simulink model "TWFL_V2"  (R2025b)
settings: Solver=daessc  StartTime=0.0  StopTime=15  RelTol=1e-3
values from neighbouring files (symbols this model uses):
  g = 9.81    [model_simplified.m]    (also in robotParams.m)
  g_fork = 2*pi*3    (= 18.8495559215)    [robotParams.m]
  g_lift = 2*pi*5    (= 31.4159265359)    [robotParams.m]
  g_reac = 2*pi*1    (= 6.28318530718)    [robotParams.m]
  Kd_fork = 100    [robotParams.m]
  Kd_lift = 50    [robotParams.m]
  Kp_fork = 200    [robotParams.m]
  Kp_lift = 200    [robotParams.m]
  Lx_b = 0.3    [robotParams.m]
  Lx_m = 0.1    [robotParams.m]
  Ly_b = 0.8    [robotParams.m]
  Ly_m = 0.3    [robotParams.m]
  Lz_b = 1    [robotParams.m]
  Lz_m = 1.5    [robotParams.m]
  M_arm_motor = 5    [robotParams.m]
  M_b = 16    [robotParams.m]
  M_fork_base = 2    [robotParams.m]
  M_m = 5    [robotParams.m]
  M_tooth = 1    [robotParams.m]
  M_w = 1    [robotParams.m]
  N = 40    [ocp_arm.m]    (also in ocp_simplified.m)
  r_w = 0.2    [model_simplified.m]    (also in robotParams.m)
  T_control = 1e-3    (= 0.001)    [robotParams.m]
  t_w = 0.05    [robotParams.m]
undefined symbols (not defined in the file or in its folder): dspblkCoreblockFVToolHelper, gcbh, Mn_33, Mn_44, X, Y, Z
libraries: sm_lib x49, nesl_utility x13, simulink x9, slpidlib x1, SignalEditorBlockLib x1
(part 3 of 3)

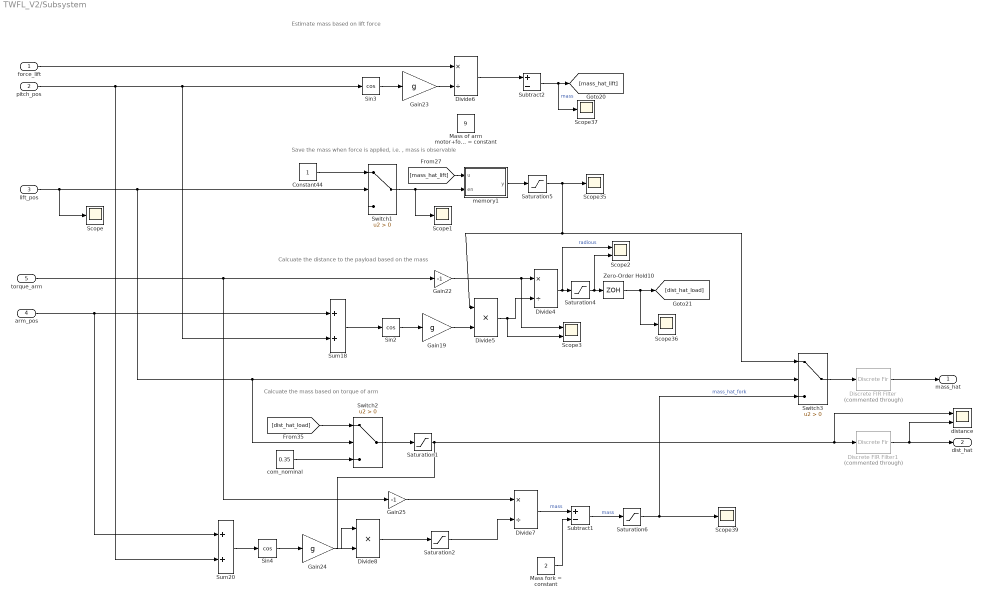
== system TWFL_V2/Subsystem ==
  note: Estimate mass based on lift force
  note: Save the mass when force is applied, i.e. , mass is observable
  note: Calcuate the distance to the payload based on the mass
  note: Calcuate the mass based on torque of arm
  force_lift : Inport
  pitch_pos : Inport  Port=2
  lift_pos : Inport  Port=3
  arm_pos : Inport  Port=4
  torque_arm : Inport  Port=5
  Constant44 : Constant
  Discrete FIR Filter : DiscreteFir  Commented=through  LoadFcn=dspblkCoreblockFVToolHelper(gcbh,'load');  Coefficients=ones(1,5000)/5000
      settings: CopyFcn=dspblkCoreblockFVToolHelper(gcbh,'copy');  DeleteFcn=dspblkCoreblockFVToolHelper(gcbh,'close');  ModelCloseFcn=dspblkCoreblockFVToolHelper(gcbh,'close');  PreSaveFcn=dspblkCoreblockFVToolHelper(gcbh,'presave');  PostSaveFcn=dspblkCoreblockFVToolHelper(gcbh,'postsave');  CloseFcn=dspblkCoreblockFVToolHelper(gcbh,'close');
  Discrete FIR Filter1 : DiscreteFir  Commented=through  LoadFcn=dspblkCoreblockFVToolHelper(gcbh,'load');  Coefficients=ones(1,500)/500
      settings: CopyFcn=dspblkCoreblockFVToolHelper(gcbh,'copy');  DeleteFcn=dspblkCoreblockFVToolHelper(gcbh,'close');  ModelCloseFcn=dspblkCoreblockFVToolHelper(gcbh,'close');  PreSaveFcn=dspblkCoreblockFVToolHelper(gcbh,'presave');  PostSaveFcn=dspblkCoreblockFVToolHelper(gcbh,'postsave');  CloseFcn=dspblkCoreblockFVToolHelper(gcbh,'close');
  Divide4 : Product  Inputs=*/
  Divide5 : Product  Inputs=**
  Divide6 : Product  Inputs=*/
  Divide7 : Product  Inputs=*/
  Divide8 : Product  Inputs=**
  Gain19 : Gain  Gain=g
  Gain22 : Gain  Gain=-1
  Gain23 : Gain  Gain=g
  Gain24 : Gain  Gain=g
  Gain25 : Gain  Gain=-1
  Mass fork = constant : Constant  Value=2
  Mass of arm motor+fork = constant : Constant  Value=9
  Saturation1 : Saturate  UpperLimit=0.6  LowerLimit=0.1
  Saturation2 : Saturate  UpperLimit=inf  LowerLimit=0.1
  Saturation4 : Saturate  UpperLimit=0.6  LowerLimit=0.1
  Saturation5 : Saturate  UpperLimit=20  LowerLimit=0.001
  Saturation6 : Saturate  UpperLimit=20  LowerLimit=0
  Scope{,1,35..37,39} (6 alike) : Scope
      Scope settings: ActiveDisplayYMinimum=0.070361077430227931  ActiveDisplayYMaximum=0.28346517515409136  DataLoggingVariableName=ScopeData8
      Scope1 settings: ActiveDisplayYMinimum=-1  ActiveDisplayYMaximum=1  DataLoggingVariableName=ScopeData23
      Scope35 settings: ActiveDisplayYMinimum=-8.2304071109691854  ActiveDisplayYMaximum=20.638497565504139  DataLoggingVariableName=ScopeData41
      Scope36 settings: ActiveDisplayYMinimum=0.4275366294753099  ActiveDisplayYMaximum=0.68738197605097551  DataLoggingVariableName=ScopeData42
      Scope37 settings: ActiveDisplayYMinimum=-38.285966258289932  ActiveDisplayYMaximum=64.906768166290135  DataLoggingVariableName=ScopeData43
      Scope39 settings: ActiveDisplayYMinimum=-0.718038981848304  ActiveDisplayYMaximum=31.278716537533729  DataLoggingVariableName=ScopeData45
  Scope2 : Scope  NumInputPorts=2
      settings: ActiveDisplayYMinimum=-736.6219251517366  ActiveDisplayYMaximum=1535.2926904846679  DataLoggingVariableName=ScopeData24
  Scope3 : Scope  NumInputPorts=2
      settings: ActiveDisplayYMinimum=69.229442757721216  ActiveDisplayYMaximum=203.32446584581058  DataLoggingVariableName=ScopeData25
  Sin2 : Trigonometry  Operator=cos
  Sin3 : Trigonometry  Operator=cos
  Sin4 : Trigonometry  Operator=cos
  Subtract1 : Sum  Inputs=+-
  Subtract2 : Sum  Inputs=+-
  Sum18 : Sum
  Sum20 : Sum
  Switch1 : Switch  Criteria=u2 > Threshold  SaturateOnIntegerOverflow=off  InputSameDT=off
  Switch2 : Switch  Criteria=u2 > Threshold  SaturateOnIntegerOverflow=off  InputSameDT=off
  Switch3 : Switch  Criteria=u2 > Threshold  SaturateOnIntegerOverflow=off  InputSameDT=off
  Zero-Order Hold10 : ZeroOrderHold  SampleTime=-1
  com_nominal : Constant  Value=0.35
  distance : Scope  NumInputPorts=2
      settings: ActiveDisplayYMinimum=0.036644537384693643  ActiveDisplayYMaximum=0.99273896289250629  DataLoggingVariableName=ScopeData47
  memory1 : MATLAB Function  TreatAsAtomicUnit=on
  mass_hat : Outport
  dist_hat : Outport  Port=2
  wires:
  Constant44/1 -> Switch1/1
  memory1/1(y) -> Saturation5/1
  pitch_pos/1 -> Sum20/2, Sin3/1, Sum18/2
  lift_pos/1 -> Scope/1, Switch1/2, Switch2/2, Switch3/2
  com_nominal/1 -> Switch2/3
  Divide5/1 -> Scope3/2, Divide4/2
  force_lift/1 -> Divide6/1
  [mass_hat_lift] -> memory1/1(u)
  Switch1/1 -> Scope1/1, memory1/2(en)
  Zero-Order Hold10/1 -> [dist_hat_load], Scope36/1
  [dist_hat_load] -> Switch2/1
  Sin4/1 -> Gain24/1
  Switch2/1 -> Saturation1/1
  Sin3/1 -> Gain23/1
  arm_pos/1 -> Sum20/1, Sum18/1
  Saturation5/1 -> Divide5/1, Switch3/1, Scope35/1
  Saturation4/1 -> Scope2/2, Zero-Order Hold10/1
  Divide4/1 -> Scope2/1, Saturation4/1  "radious"
  torque_arm/1 -> Gain22/1, Gain25/1
  Sum20/1 -> Sin4/1
  Saturation6/1 -> Switch3/3, Scope39/1  "mass_hat_fork"
  Sin2/1 -> Gain19/1
  Switch3/1 -> Discrete FIR Filter/1
  Gain25/1 -> Divide7/1
  Divide6/1 -> Subtract2/1
  Gain22/1 -> Scope3/1, Divide4/1
  Divide7/1 -> Subtract1/1  "mass"
  Gain24/1 -> Divide8/1
  Divide8/1 -> Saturation2/1
  Sum18/1 -> Sin2/1
  Gain19/1 -> Divide5/2
  Subtract2/1 -> Scope37/1, [mass_hat_lift]  "mass"
  Gain23/1 -> Divide6/2
  Mass fork = constant/1 -> Subtract1/2
  Subtract1/1 -> Saturation6/1  "mass"
  Discrete FIR Filter1/1 -> distance/2, dist_hat/1
  Discrete FIR Filter/1 -> mass_hat/1
  Saturation1/1 -> Discrete FIR Filter1/1, distance/1, Divide8/2
  Saturation2/1 -> Divide7/2

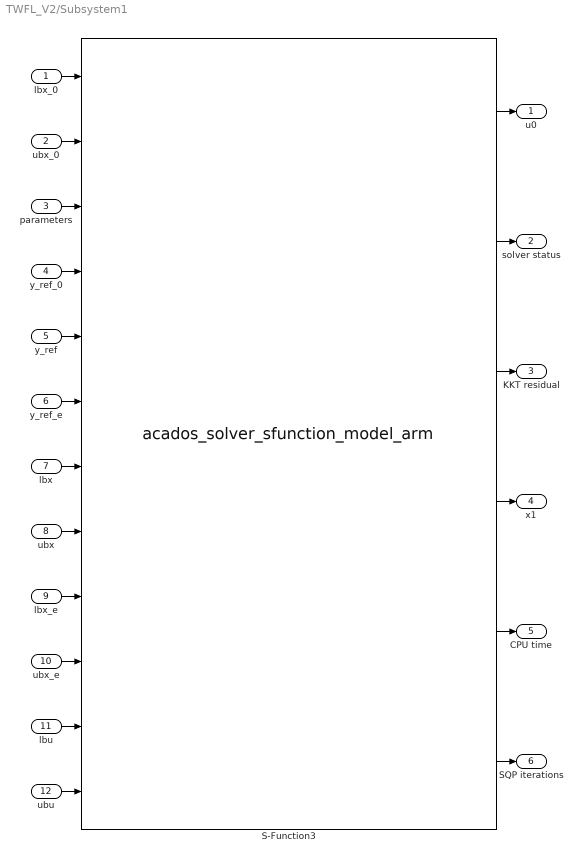
== system TWFL_V2/Subsystem1 ==
  lbx_0 : Inport
  ubx_0 : Inport  Port=2
  parameters : Inport  Port=3
  y_ref_0 : Inport  Port=4
  y_ref : Inport  Port=5
  y_ref_e : Inport  Port=6
  lbx : Inport  Port=7
  ubx : Inport  Port=8
  lbx_e : Inport  Port=9
  ubx_e : Inport  Port=10
  lbu : Inport  Port=11
  ubu : Inport  Port=12
  S-Function3 : S-Function  FunctionName=acados_solver_sfunction_model_arm  SFunctionDeploymentMode=off  EnableBusSupport=off
  u0 : Outport
  solver status : Outport  Port=2
  KKT residual : Outport  Port=3
  x1 : Outport  Port=4
  CPU time : Outport  Port=5
  SQP iterations : Outport  Port=6
  wires:
  y_ref/1 -> S-Function3/5
  lbx_e/1 -> S-Function3/9
  ubx_0/1 -> S-Function3/2
  lbx_0/1 -> S-Function3/1
  lbu/1 -> S-Function3/11
  lbx/1 -> S-Function3/7
  parameters/1 -> S-Function3/3
  y_ref_e/1 -> S-Function3/6
  ubx/1 -> S-Function3/8
  y_ref_0/1 -> S-Function3/4
  S-Function3/1 -> u0/1
  ubu/1 -> S-Function3/12
  S-Function3/3 -> KKT residual/1
  ubx_e/1 -> S-Function3/10
  S-Function3/2 -> solver status/1
  S-Function3/6 -> SQP iterations/1
  S-Function3/4 -> x1/1
  S-Function3/5 -> CPU time/1

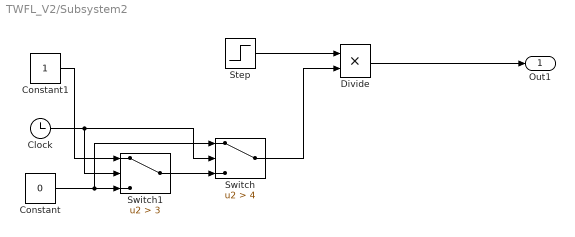
== system TWFL_V2/Subsystem2 ==
  Clock : Clock
      settings: Decimation=7
  Constant : Constant  Value=0
  Constant1 : Constant
  Divide : Product  Inputs=**
  Step : Step  After=30  SampleTime=0
  Switch : Switch  Criteria=u2 > Threshold  Threshold=4  SaturateOnIntegerOverflow=off  InputSameDT=off
  Switch1 : Switch  Criteria=u2 > Threshold  Threshold=3  SaturateOnIntegerOverflow=off  InputSameDT=off
  Out1 : Outport
  wires:
  Switch/1 -> Divide/2
  Switch1/1 -> Switch/3
  Clock/1 -> Switch1/2, Switch/2
  Constant/1 -> Switch/1, Switch1/3
  Constant1/1 -> Switch1/1
  Step/1 -> Divide/1
  Divide/1 -> Out1/1

== system TWFL_V2/Calculations/myDerivative1 ==
  In1 : Inport
  Delay3 : Delay  DelayLength=1  InputProcessing=Columns as channels (frame based)
  Gain23 : Gain  Gain=1/T_control
  Subtract2 : Sum  Inputs=+-
  Out1 : Outport
  wires:
  Gain23/1 -> Out1/1
  Subtract2/1 -> Gain23/1
  Delay3/1 -> Subtract2/2
  In1/1 -> Subtract2/1, Delay3/1

== system TWFL_V2/Calculations/myDerivative2 ==
  In1 : Inport
  Delay3 : Delay  DelayLength=1  InputProcessing=Columns as channels (frame based)
  Gain23 : Gain  Gain=1/T_control
  Subtract2 : Sum  Inputs=+-
  Out1 : Outport
  wires:
  Gain23/1 -> Out1/1
  Subtract2/1 -> Gain23/1
  Delay3/1 -> Subtract2/2
  In1/1 -> Subtract2/1, Delay3/1

== system TWFL_V2/Calculations/myDerivative3 ==
  In1 : Inport
  Delay3 : Delay  DelayLength=1  InputProcessing=Columns as channels (frame based)
  Gain23 : Gain  Gain=1/T_control
  Subtract2 : Sum  Inputs=+-
  Out1 : Outport
  wires:
  In1/1 -> Delay3/1, Subtract2/1
  Delay3/1 -> Subtract2/2
  Subtract2/1 -> Gain23/1
  Gain23/1 -> Out1/1

== system TWFL_V2/Calculations/myDerivative4 ==
  In1 : Inport
  Delay3 : Delay  DelayLength=1  InputProcessing=Columns as channels (frame based)
  Gain23 : Gain  Gain=1/T_control
  Subtract2 : Sum  Inputs=+-
  Out1 : Outport
  wires:
  Gain23/1 -> Out1/1
  Subtract2/1 -> Gain23/1
  Delay3/1 -> Subtract2/2
  In1/1 -> Subtract2/1, Delay3/1

== system TWFL_V2/Calculations/myDerivative5 ==
  In1 : Inport
  Delay3 : Delay  DelayLength=1  InputProcessing=Columns as channels (frame based)
  Gain23 : Gain  Gain=1/T_control
  Subtract2 : Sum  Inputs=+-
  Out1 : Outport
  wires:
  In1/1 -> Delay3/1, Subtract2/1
  Delay3/1 -> Subtract2/2
  Subtract2/1 -> Gain23/1
  Gain23/1 -> Out1/1

== matlab function TWFL_V2/Subsystem/memory1 ==
  settings: updateMethod=DISCRETE
  data: u input; y output; en input
function y = fcn(u,en)
persistent mem
if isempty(mem)
    mem = 0; % valor inicial
end
if en
    mem = u;
end
y = mem;
end

== stateflow chart TWFL_V2/Chart ==
  settings: updateMethod=DISCRETE  sampleTime=1e-3
  state Init
    velocity_out = 0;
  state Move
    velocity_out = velocity_in;
  state Load
    velocity_out = 0;
  state Collision
    velocity_out = -1;
  state Init1
    velocity_out = 0;
  (default) -> Init
  Init -> Move [order 2] : [move == 1]
  Init -> Load [order 1] : [load==1]
  Move -> Load [order 2] : [load==1]
  Load -> Move : [move == 1]
  Move -> Collision [order 1] : [collision==1]
  Collision -> Init1 : after(1,sec)
  data: collision input; velocity_out output; move input; load input; velocity_in input

== matlab function TWFL_V2/MATLAB Function1 ==
  settings: updateMethod=DISCRETE  sampleTime=T_control
  data: m_hat input; cdg output; pos_lift input; d_hat input; I_total output; M_b parameter
function [cdg, I_total] = new_cdg_and_inertia(m_hat, pos_lift, d_hat, M_b)
%#codegen
% Compute total center of gravity and equivalent inertia (Y axis)
% Suitable for Simulink / code generation

% -------------------------------
% Fixed model parameters
% -------------------------------
m = [M_b;
     5.0;
     5.0;
     2.0;
     m_hat];

x = [ 0.0;
     -0.15;
     -0.10;
      0.30;
     -0.10 + d_hat];

z = [1/2;
     1.20 + pos_lift;
     1.05 + pos_lift;
     1.05 + pos_lift;
     1.05 + pos_lift];

I_y = [1.4533;
       0.9417;
       0.1531;
       0.0300;
       0.0000];

% -------------------------------
% Total mass
% -------------------------------
M = m(1) + m(2) + m(3) + m(4) + m(5);

% -------------------------------
% Center of gravity
% -------------------------------
x_G = (m(1)*x(1) + m(2)*x(2) + m(3)*x(3) + m(4)*x(4) + m(5)*x(5)) / M;
z_G = (m(1)*z(1) + m(2)*z(2) + m(3)*z(3) + m(4)*z(4) + m(5)*z(5)) / M;

cdg = [x_G; z_G];   % 2x1 vector (Simulink-friendly)

% -------------------------------
% Steiner inertia
% -------------------------------
dx1 = x(1) - x_G; dz1 = z(1) - z_G;
dx2 = x(2) - x_G; dz2 = z(2) - z_G;
dx3 = x(3) - x_G; dz3 = z(3) - z_G;
dx4 = x(4) - x_G; dz4 = z(4) - z_G;
dx5 = x(5) - x_G; dz5 = z(5) - z_G;

I_total = ...
    I_y(1) + m(1)*(dx1*dx1 + dz1*dz1) + ...
    I_y(2) + m(2)*(dx2*dx2 + dz2*dz2) + ...
    I_y(3) + m(3)*(dx3*dx3 + dz3*dz3) + ...
    I_y(4) + m(4)*(dx4*dx4 + dz4*dz4) + ...
    I_y(5) + m(5)*(dx5*dx5 + dz5*dz5);

end
